simulink model "sensor_frequency_sweep"  (R2022a)
settings: Solver=VariableStepAuto  StartTime=0.0  StopTime=Tsim  RelTol=1e-3
values from neighbouring files (symbols this model uses):
  Ain = 1    [run_frequency_sweep.m]
  k = 1.2    [run_frequency_sweep.m]
  omega = omega_values(i)    [run_frequency_sweep.m]
  r = 0.2    [run_frequency_sweep.m]
  x0 = 0    [measure_frequency_point.m]
  y0 = 0    [measure_frequency_point.m]
settings Model: Creator=HJL  LastModifiedBy=HJL

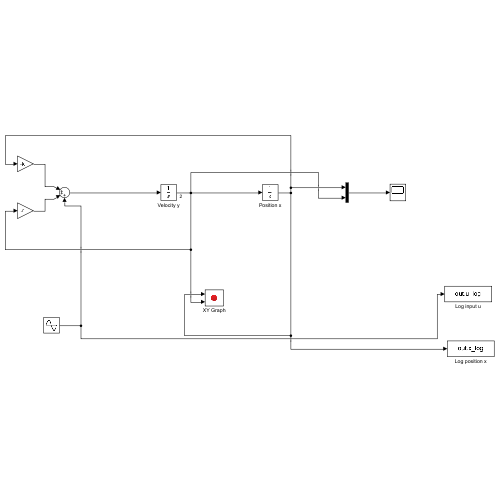
[thumbnail: Simulink's stored preview of the top-level diagram]
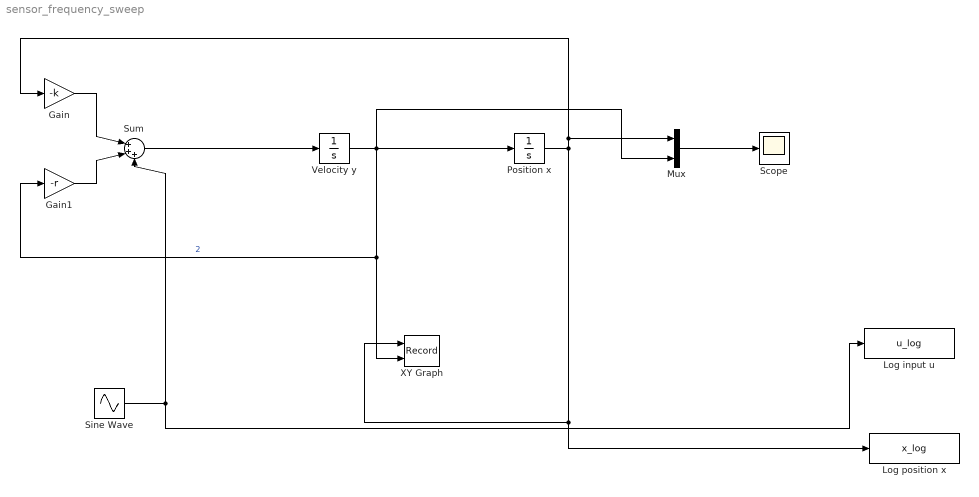
== system sensor_frequency_sweep ==
  Gain : Gain  Gain=-k
  Gain1 : Gain  Gain=-r
  Log input u : ToWorkspace  VariableName=u_log  SaveFormat=Timeseries  SampleTime=-1
  Log position x : ToWorkspace  VariableName=x_log  SaveFormat=Timeseries  SampleTime=-1
  Mux : Mux  Inputs=2
  Position x : Integrator  InitialCondition=x0
  Scope : Scope
  Sine Wave : Sin  Amplitude=Ain  Frequency=omega  SampleTime=0
  Sum : Sum  Inputs=|+++
  Velocity y : Integrator  InitialCondition=y0
  XY Graph : Record  FileSettingsInternal="{\"entries\":[{\"content\":{\"excelSettings\":{\"content\":{},\"type\":\"Streamout.ExcelSettings\"}},\"type\":\"Streamout.FileSettingStorage\",\"uuid\":\"6343d1be-610d-42c7-8c70-786c6973f6e9\"}],\"packageUris\":[\"http://schema.mathworks.com/mf0/streamout_blocks/R2020a\"],\"version\":\"1.0\"}"  Layout=[1 1]  SignalsInternal="{\"entries\":[{\"content\":{\"signals\":[{\"content\":{\"blockPath\":[\"sensor_frequency_sweep/XY Graph\"],\"channel\":[],\"dimensions\":[1],\"domain\":\"sensor_frequency_sweep/XY Graph\",\"lineColor\":\"#a2142f\",\"plots\":[1],\"port\":1,\"sid\":[\"\"],\"signalID\":2056,\"signalName\":\"Position x\"},\"type\":\"RecordBlkView.Signal\",\"uuid\":\"f42989cf-bf6a-4fc2-87cf-9eefce40ceb0\"},{\"content\":{\"blockPath\":[\"sensor_frequency_sweep/XY Graph\"],\"channel\":[],\"dimensions\":[1],\"domain\":\"sensor_frequency_sweep/XY Graph\",\"lineColor\":\"#139fff\",\"plots\":[1],\"port\":2,\"sid\":[\"\"],\"signalID\":2060,\"signalName\":\"2\"},\"type\":\"RecordBlkView.Signal\",\"uuid\":\"c829b593-de60-4810-8f96-432884258040\"}]},\"type\":\"RecordBlkView.InputSignals\",\"uuid\":\"330dddc5-a5ef-4232-8ce2-4c0c653d9134\"}],\"packageUris\":[\"http://schema.mathworks.com/mf0/streamout_blocks/R2020a\"],\"version\":\"1.0\"}"  VisualizationBindings="{\"xyplotplugin\":{\"info\":[{\"series\":[{\"bindingParametersList\":[{\"parameter\":\"X-Axis\",\"signalID\":2056,\"signalName\":\"Position x\"},{\"parameter\":\"Y-Axis\",\"signalID\":2060,\"signalName\":\"2\"}],\"seriesID\":4493}],\"subplotID\":1}]}}"  CompatibilityTag=XY
  wires:
  Gain1/1 -> Sum/2
  Gain/1 -> Sum/1
  Sum/1 -> Velocity y/1
  Position x/1 -> Mux/1, Gain/1, Log position x/1, XY Graph/1
  Velocity y/1 -> XY Graph/2, Gain1/1, Mux/2, Position x/1  "2"
  Mux/1 -> Scope/1
  Sine Wave/1 -> Sum/3, Log input u/1
